simulink model "MCU_Input"  (R2022b)
settings: Solver=FixedStepDiscrete  StartTime=0.0  StopTime=10.0  FixedStep=1e-4  RelTol=1e-3
values from neighbouring files (symbols this model uses):
  C_ADC_Acc1Offset_i32 = 0.0    [MCU_Input_Sldd.sldd]    (also in MCU_Input_Sldd_objects.m = myPackage.Parameter)
  C_ADC_BrakeOffset_i32 = 0.0    [MCU_Input_Sldd.sldd]    (also in MCU_Input_Sldd_objects.m = myPackage.Parameter)
  C_ADC_HSTempGain_f32 = 0.0    [MCU_Input_Sldd.sldd]    (also in MCU_Input_Sldd_objects.m = myPackage.Parameter)
  C_ADC_HSTempOffset_i32 = 0.0    [MCU_Input_Sldd.sldd]    (also in MCU_Input_Sldd_objects.m = myPackage.Parameter)
  C_ADC_IdcOffset_i32 = 0.0    [MCU_Input_Sldd.sldd]    (also in MCU_Input_Sldd_objects.m = myPackage.Parameter)
  C_ADC_IGBTTable_i16 = 0.0    [MCU_Input_Sldd.sldd]    (also in MCU_Input_Sldd_objects.m = myPackage.Parameter)
  C_ADC_IGBTTempGain_f32 = 0.0    [MCU_Input_Sldd.sldd]    (also in MCU_Input_Sldd_objects.m = myPackage.Parameter)
  C_ADC_IGBTTempOffset_i32 = 0.0    [MCU_Input_Sldd.sldd]    (also in MCU_Input_Sldd_objects.m = myPackage.Parameter)
  C_ADC_MotorTemp1Gain_f32 = 0.0    [MCU_Input_Sldd.sldd]    (also in MCU_Input_Sldd_objects.m = myPackage.Parameter)
  C_ADC_MotorTemp1Offset_i32 = 0.0    [MCU_Input_Sldd.sldd]    (also in MCU_Input_Sldd_objects.m = myPackage.Parameter)
  C_ADC_MotorTempTable_i16 = 0.0    [MCU_Input_Sldd.sldd]    (also in MCU_Input_Sldd_objects.m = myPackage.Parameter)
  C_ADC_P12VOffset_i32 = 0.0    [MCU_Input_Sldd.sldd]    (also in MCU_Input_Sldd_objects.m = myPackage.Parameter)
  C_ADC_P15VOffset_i32 = 0.0    [MCU_Input_Sldd.sldd]    (also in MCU_Input_Sldd_objects.m = myPackage.Parameter)
  C_ADC_P5VOffset_i32 = 0.0    [MCU_Input_Sldd.sldd]    (also in MCU_Input_Sldd_objects.m = myPackage.Parameter)
  C_DCCurrent_DrvCoeff_f32 = 0.0    [MCU_Input_Sldd.sldd]    (also in MCU_Input_Sldd_objects.m = myPackage.Parameter)
  C_DCCurrent_GenCoeff_f32 = 0.0    [MCU_Input_Sldd.sldd]    (also in MCU_Input_Sldd_objects.m = myPackage.Parameter)
  C_Encoder_CurrentAdder_f32 = 0.0    [MCU_Input_Sldd.sldd]    (also in MCU_Input_Sldd_objects.m = myPackage.Parameter)
  C_Encoder_WaitTime_f32 = 0.0    [MCU_Input_Sldd.sldd]    (also in MCU_Input_Sldd_objects.m = myPackage.Parameter)
  C_Input_EncErr_u8 = 0.0    [MCU_Input_Sldd.sldd]    (also in MCU_Input_Sldd_objects.m = myPackage.Parameter)
  C_Rotate_RotateBits_u8 = 0.0    [MCU_Input_Sldd.sldd]    (also in MCU_Input_Sldd_objects.m = myPackage.Parameter)
  C_Rotate_SetAngle_u16 = 0.0    [MCU_Input_Sldd.sldd]    (also in MCU_Input_Sldd_objects.m = myPackage.Parameter)
  C_Rotate_SetAngleFlg_u8 = 0.0    [MCU_Input_Sldd.sldd]    (also in MCU_Input_Sldd_objects.m = myPackage.Parameter)
  C_SelfCheck_AvgCntSet_u16 = 0.0    [MCU_Input_Sldd.sldd]    (also in MCU_Input_Sldd_objects.m = myPackage.Parameter)
  C_SelfCheck_DelayTimeSet_u16 = 0.0    [MCU_Input_Sldd.sldd]    (also in MCU_Input_Sldd_objects.m = myPackage.Parameter)
  C_SelfCheck_IaoffsetDownLimt_u16 = 0.0    [MCU_Input_Sldd.sldd]    (also in MCU_Input_Sldd_objects.m = myPackage.Parameter)
  C_SelfCheck_IaoffsetUpLimt_u16 = 0.0    [MCU_Input_Sldd.sldd]    (also in MCU_Input_Sldd_objects.m = myPackage.Parameter)
  C_SelfCheck_IboffsetDownLimt_u16 = 0.0    [MCU_Input_Sldd.sldd]    (also in MCU_Input_Sldd_objects.m = myPackage.Parameter)
  C_SelfCheck_IboffsetUpLimt_u16 = 0.0    [MCU_Input_Sldd.sldd]    (also in MCU_Input_Sldd_objects.m = myPackage.Parameter)
  C_SelfCheck_IcoffsetDownLimt_u16 = 0.0    [MCU_Input_Sldd.sldd]    (also in MCU_Input_Sldd_objects.m = myPackage.Parameter)
  C_SelfCheck_IcoffsetUpLimt_u16 = 0.0    [MCU_Input_Sldd.sldd]    (also in MCU_Input_Sldd_objects.m = myPackage.Parameter)
  C_SelfCheck_OffsetUnCal_u8 = 0.0    [MCU_Input_Sldd.sldd]    (also in MCU_Input_Sldd_objects.m = myPackage.Parameter)
undefined symbols (not defined in the file or in its folder): AB_SAMPLE, ABC_SAMPLE, AC_SAMPLE, ANALOG, BC_SAMPLE, cAgeingMode, cParaRecogMode, cVvvfOpenMode, ParamCfg_AdAcc1K_u16, ParamCfg_AdBrakeK_u16, ParamCfg_AdIaK_u16, ParamCfg_AdIbK_u16, ParamCfg_AdIcK_u16, ParamCfg_AdKeyK_u16, ParamCfg_AdP12vK_u16, ParamCfg_AdP15vK_u16, ParamCfg_AdP5vK_u16, ParamCfg_AdUdcK_u16, ParamCfg_AdVonK_u16, ParamCfg_Avgcnt_u16, ParamCfg_BaseCur_u16, ParamCfg_BaseUdc_u16, ParamCfg_CommandSource_u16, ParamCfg_MaxSpeed_u16, ParamCfg_MotorNp_u16, ParamCfg_PosInit_u16, ParamCfg_PowerMax_u16, ParamCfg_PwmFreqLow_u16, ParamCfg_RotateDir_u16, ParamCfg_RotateNp_u16, ParamCfg_SampleMode_u16, ParamCfg_SensorSpeed_u16, ParamCfg_SmoPllKi_u16, ParamCfg_SmoPllKp_u16, ParamCfg_Stage_u16, ParamCfg_ThetaGain_u16, ParamCfg_UdcDefValue_u16, POWER_ON, STANDBY
libraries: simulink x41, YS_UserDefined_Library x4
(part 3 of 5)

== system MCU_Input/Input_100us/DCCurrent_100us/DcCurrentCal/FirstOrder_LPF_Calc ==
  Xn : Inport
  Add : Sum
  Compare To Constant : simulink/Logic and Bit Operations/Compare To Constant  relop=<  const=1  OutDataTypeStr=boolean
  Constant : Constant  Value=0.01  OutDataTypeStr=single
  Constant1 : Constant  OutDataTypeStr=single
  Minus : Sum  Inputs=+-
  Minus1 : Sum  Inputs=-+
  Product : Product
  Product1 : Product
  Switch : Switch  Criteria=u2 > Threshold  SaturateOnIntegerOverflow=off  InputSameDT=off
  Unit Delay : UnitDelay  SampleTime=-1  HasFrameUpgradeWarning=on
  Yn : Outport
  wires:
  Switch/1 -> Unit Delay/1, Yn/1
  Unit Delay/1 -> Product1/2, Minus/2  "Yn_1"
  Xn/1 -> Minus/1, Product/1, Switch/1
  Minus/1 -> Compare To Constant/1
  Compare To Constant/1 -> Switch/2
  Constant/1 -> Minus1/1, Product/2
  Product/1 -> Add/1
  Constant1/1 -> Minus1/2
  Minus1/1 -> Product1/1
  Product1/1 -> Add/2
  Add/1 -> Switch/3

== system MCU_Input/Input_100us/DCCurrent_100us/DcCurrentCal/RandCurGen ==
  Add : Sum
  Compare To Constant : simulink/Logic and Bit Operations/Compare To Constant  relop=>=  const=41  OutDataTypeStr=boolean
  Constant : Constant  OutDataTypeStr=uint8
  RandCurArray : Constant  Value=[1, 7, 5, 2, 4, 5, 8, 6, 3, 5, 1, 10, 7, 5, 0, 2, 4, 5, 8, 6, 3, 8, 6, 3, 5, 1, 10, 7, 5, 2, 10, 7, 5, 0, 2, 4, 5, 8, 6, 3, 8]  OutDataTypeStr=uint16
  Selector : Selector  InputPortWidth=41  IndexOptions=Index vector (port)  Indices=[1 3]  OutputSizes=1
  Switch : Switch  Criteria=u2 ~= 0  SaturateOnIntegerOverflow=off  InputSameDT=off
  Unit Delay : UnitDelay  SampleTime=-1  HasFrameUpgradeWarning=on
  RandCur : Outport
  wires:
  Add/1 -> Selector/2, Unit Delay/1
  Constant/1 -> Add/1, Switch/1
  Compare To Constant/1 -> Switch/2
  Unit Delay/1 -> Switch/3, Compare To Constant/1
  Switch/1 -> Add/2
  RandCurArray/1 -> Selector/1
  Selector/1 -> RandCur/1

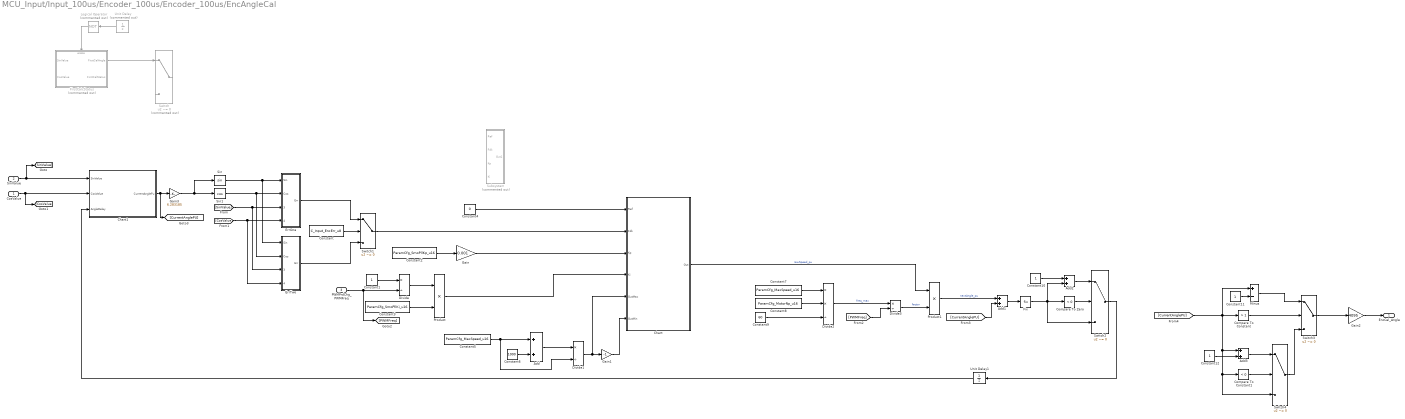
== system MCU_Input/Input_100us/Encoder_100us/Encoder_100us/EncAngleCal ==
  CosValue : Inport
  SinValue : Inport  Port=2
  PWMPrdChg_PWMFreq : Inport  Port=3
  Add : Sum
  Add1 : Sum  OutDataTypeStr=single
  Add2 : Sum
  Add3 : Sum
  Chart : Stateflow chart  TreatAsAtomicUnit=on
  Chart1 : Stateflow chart  TreatAsAtomicUnit=on
  Compare To Constant : simulink/Logic and Bit Operations/Compare To Constant  relop=>  const=1  OutDataTypeStr=boolean
  Compare To Constant1 : simulink/Logic and Bit Operations/Compare To Constant  relop=<  const=0  OutDataTypeStr=boolean
  Compare To Zero : simulink/Logic and Bit Operations/Compare To Zero  relop=<  OutDataTypeStr=boolean
  Constant : Constant  Value=C_Input_EncErr_u8
  Constant{1,10..12} (4 alike) : Constant  OutDataTypeStr=single
  Constant2 : Constant  Value=ParamCfg_SmoPllKp_u16
  Constant3 : Constant  Value=ParamCfg_SmoPllKi_u16
  Constant4 : Constant  Value=0  OutDataTypeStr=single
  Constant5 : Constant  Value=ParamCfg_MaxSpeed_u16
  Constant6 : Constant  Value=1000  OutDataTypeStr=single
  Constant7 : Constant  Value=ParamCfg_MaxSpeed_u16
  Constant8 : Constant  Value=ParamCfg_MotorNp_u16
  Constant9 : Constant  Value=60  OutDataTypeStr=single
  Divide : Product  Inputs=*/  OutDataTypeStr=single
  Divide1 : Product  Inputs=*/
  Divide2 : Product  Inputs=**/
  Divide3 : Product  Inputs=*/
  ErrOne : Subsystem
  ErrTwo : Subsystem
  FirstCalcStatus : Subsystem  Commented=on
  Fix : Rounding  Operator=fix
  Gain : Gain  Gain=0.001  ParamDataTypeStr=single  OutDataTypeStr=single
  Gain1 : Gain  Gain=-1  ParamDataTypeStr=single  OutDataTypeStr=single
  Gain2 : Gain  Gain=4095  ParamDataTypeStr=uint16  OutDataTypeStr=uint16
  Gain3 : Gain  Gain=6.283185  ParamDataTypeStr=single  OutDataTypeStr=single
      settings: AttributesFormatString=%<Gain>
  Logical Operator : Logic  Commented=on  Operator=NOT  AllPortsSameDT=off  OutDataTypeStr=boolean
  Minus : Sum  Inputs=+-
  Product : Product
  Product1 : Product
  Sin : Trigonometry
  Sin1 : Trigonometry  Operator=cos
  Subsystem : Subsystem  Commented=on
  Switch : Switch  Commented=on  Criteria=u2 ~= 0  SaturateOnIntegerOverflow=off  InputSameDT=off
  Switch{1..4} (4 alike) : Switch  Criteria=u2 ~= 0  SaturateOnIntegerOverflow=off  InputSameDT=off
  Unit Delay : UnitDelay  Commented=on  SampleTime=-1  HasFrameUpgradeWarning=on
  Unit Delay1 : UnitDelay  SampleTime=-1  HasFrameUpgradeWarning=on
  EncCal_Angle : Outport
  wires:
  SinValue/1 -> [SinValue], Chart1/1(SinValue)
  CosValue/1 -> Chart1/2(CosValue), [CosValue]
  Chart1/1(CurrentAnglePu) -> [CurrentAnglePU], Gain3/1
  Unit Delay/1 -> Logical Operator/1
  Logical Operator/1 -> FirstCalcStatus/Enable
  FirstCalcStatus/1(FirstCalAngle) -> Switch/1
  Sin/1 -> ErrTwo/1(Sin), ErrOne/1(Sin)
  Sin1/1 -> ErrTwo/2(Cos), ErrOne/2(Cos)
  [SinValue] -> ErrTwo/3(SinValue), ErrOne/3(SinValue)
  [CosValue] -> ErrTwo/4(CosValue), ErrOne/4(CosValue)
  Constant/1 -> Switch1/2
  ErrOne/1(Err) -> Switch1/1
  ErrTwo/1(Err) -> Switch1/3
  PWMPrdChg_PWMFreq/1 -> [PWMFreq], Divide/2
  Constant1/1 -> Divide/1
  Constant2/1 -> Gain/1
  Divide/1 -> Product/1
  Constant3/1 -> Product/2
  Constant4/1 -> Chart/1(Ref)
  Switch1/1 -> Chart/2(Fdk)
  Gain/1 -> Chart/3(Kp)
  Product/1 -> Chart/4(Ki)
  Constant6/1 -> Add/2
  Divide1/1 -> Chart/5(OutMax), Gain1/1
  Constant5/1 -> Add/1, Divide1/2
  Add/1 -> Divide1/1
  Gain1/1 -> Chart/6(OutMin)
  Chart/1(Out) -> Product1/1  "rawSpeed_pu"
  Constant7/1 -> Divide2/1
  Constant8/1 -> Divide2/2
  Constant9/1 -> Divide2/3
  Divide2/1 -> Divide3/1  "freq_max"
  [PWMFreq] -> Divide3/2
  Divide3/1 -> Product1/2  "factor"
  Product1/1 -> Add1/1  "nextAngle_pu"
  Add1/1 -> Fix/1
  Unit Delay1/1 -> Chart1/3(AngleDelay)
  Fix/1 -> Add2/2, Switch2/3, Compare To Zero/1
  Compare To Zero/1 -> Switch2/2
  Add2/1 -> Switch2/1
  Constant10/1 -> Add2/1
  [CurrentAnglePU] -> Compare To Constant/1, Switch4/3, Compare To Constant1/1, Add3/1, Minus/1
  Compare To Constant/1 -> Switch3/2
  Constant11/1 -> Minus/2
  Minus/1 -> Switch3/1
  Switch4/1 -> Switch3/3
  Compare To Constant1/1 -> Switch4/2
  Add3/1 -> Switch4/1
  Constant12/1 -> Add3/2
  Switch3/1 -> Gain2/1
  Gain2/1 -> EncCal_Angle/1
  Gain3/1 -> Sin/1, Sin1/1
  [CurrentAnglePU] -> Add1/2
  Switch2/1 -> Unit Delay1/1

== system MCU_Input/Input_100us/Encoder_100us/Encoder_100us/EncCalibCal/AmpCos ==
  CosRaw : Inport  OutDataTypeStr=uint16  PortDimensions=1
  f : TriggerPort  TriggerType=function-call  VariantControl=(inherit)
      settings: CopyFcn=Stateflow.SLINSF.SimulinkMan.removeBlockPreDeleteFcn  PreDeleteFcn=Stateflow.SLINSF.SimulinkMan.unsafePredeleteFcn
  Data Store Read : DataStoreRead  DataStoreName=CosMin  IndexOptions=Index vector (dialog)  Indices=1  OutputSizes=1
  Data Store Read1 : DataStoreRead  DataStoreName=CosMax  IndexOptions=Index vector (dialog)  Indices=1  OutputSizes=1
  Data Store Write : DataStoreWrite  DataStoreName=CosMax  IndexOptions=Index vector (dialog)  Indices=1  OutputSizes=1
  Data Store Write1 : DataStoreWrite  DataStoreName=CosMin  IndexOptions=Index vector (dialog)  Indices=1  OutputSizes=1
  Gain : Gain  Gain=0.5  ParamDataTypeStr=single  OutDataTypeStr=single
  Minus : Sum  Inputs=+-
  Relational Operator : RelationalOperator  Operator=>  OutDataTypeStr=boolean  RndMeth=Simplest  InputSameDT=off
  Relational Operator1 : RelationalOperator  Operator=<  OutDataTypeStr=boolean  RndMeth=Simplest  InputSameDT=off
  Switch : Switch  Criteria=u2 ~= 0  SaturateOnIntegerOverflow=off  InputSameDT=off
  Switch1 : Switch  Criteria=u2 ~= 0  SaturateOnIntegerOverflow=off  InputSameDT=off
  CosAmp : Outport  OutDataTypeStr=single
  wires:
  CosRaw/1 -> Switch1/1, Relational Operator1/1, Switch/1, Relational Operator/1
  Data Store Read1/1 -> Switch/3, Relational Operator/2
  Relational Operator/1 -> Switch/2
  Switch/1 -> Minus/1, Data Store Write/1
  Data Store Read/1 -> Switch1/3, Relational Operator1/2
  Relational Operator1/1 -> Switch1/2
  Switch1/1 -> Minus/2, Data Store Write1/1
  Minus/1 -> Gain/1
  Gain/1 -> CosAmp/1

== system MCU_Input/Input_100us/Encoder_100us/Encoder_100us/EncCalibCal/AmpSin ==
  SinRaw : Inport  OutDataTypeStr=uint16  PortDimensions=1
  f : TriggerPort  TriggerType=function-call  VariantControl=(inherit)
      settings: CopyFcn=Stateflow.SLINSF.SimulinkMan.removeBlockPreDeleteFcn  PreDeleteFcn=Stateflow.SLINSF.SimulinkMan.unsafePredeleteFcn
  Data Store Read : DataStoreRead  DataStoreName=SinMin  IndexOptions=Index vector (dialog)  Indices=1  OutputSizes=1
  Data Store Read1 : DataStoreRead  DataStoreName=SinMax  IndexOptions=Index vector (dialog)  Indices=1  OutputSizes=1
  Data Store Write : DataStoreWrite  DataStoreName=SinMax  IndexOptions=Index vector (dialog)  Indices=1  OutputSizes=1
  Data Store Write1 : DataStoreWrite  DataStoreName=SinMin  IndexOptions=Index vector (dialog)  Indices=1  OutputSizes=1
  Gain : Gain  Gain=0.5  ParamDataTypeStr=single  OutDataTypeStr=single
  Minus : Sum  Inputs=+-  AccumDataTypeStr=uint16  OutDataTypeStr=uint16
  Relational Operator : RelationalOperator  Operator=>  OutDataTypeStr=boolean  RndMeth=Simplest  InputSameDT=off
  Relational Operator1 : RelationalOperator  Operator=<  OutDataTypeStr=boolean  RndMeth=Simplest  InputSameDT=off
  Switch : Switch  Criteria=u2 ~= 0  SaturateOnIntegerOverflow=off  InputSameDT=off
  Switch1 : Switch  Criteria=u2 ~= 0  SaturateOnIntegerOverflow=off  InputSameDT=off
  SinAmp : Outport  OutDataTypeStr=single  PortDimensions=1
  wires:
  SinRaw/1 -> Switch1/1, Relational Operator1/1, Switch/1, Relational Operator/1
  Data Store Read1/1 -> Switch/3, Relational Operator/2
  Relational Operator/1 -> Switch/2
  Switch/1 -> Minus/1, Data Store Write/1
  Data Store Read/1 -> Switch1/3, Relational Operator1/2
  Relational Operator1/1 -> Switch1/2
  Switch1/1 -> Minus/2, Data Store Write1/1
  Minus/1 -> Gain/1
  Gain/1 -> SinAmp/1

== system MCU_Input/Input_100us/Encoder_100us/Encoder_100us/EncCalibCal1/AmpCos ==
  CosRaw : Inport  OutDataTypeStr=uint16  PortDimensions=1
  f : TriggerPort  TriggerType=function-call  VariantControl=(inherit)
      settings: CopyFcn=Stateflow.SLINSF.SimulinkMan.removeBlockPreDeleteFcn  PreDeleteFcn=Stateflow.SLINSF.SimulinkMan.unsafePredeleteFcn
  Data Store Read : DataStoreRead  DataStoreName=CosMin  IndexOptions=Index vector (dialog)  Indices=1  OutputSizes=1
  Data Store Read1 : DataStoreRead  DataStoreName=CosMax  IndexOptions=Index vector (dialog)  Indices=1  OutputSizes=1
  Data Store Write : DataStoreWrite  DataStoreName=CosMax  IndexOptions=Index vector (dialog)  Indices=1  OutputSizes=1
  Data Store Write1 : DataStoreWrite  DataStoreName=CosMin  IndexOptions=Index vector (dialog)  Indices=1  OutputSizes=1
  Gain : Gain  Gain=0.5  ParamDataTypeStr=single  OutDataTypeStr=single
  Minus : Sum  Inputs=+-
  Relational Operator : RelationalOperator  Operator=>  OutDataTypeStr=boolean  RndMeth=Simplest  InputSameDT=off
  Relational Operator1 : RelationalOperator  Operator=<  OutDataTypeStr=boolean  RndMeth=Simplest  InputSameDT=off
  Switch : Switch  Criteria=u2 ~= 0  SaturateOnIntegerOverflow=off  InputSameDT=off
  Switch1 : Switch  Criteria=u2 ~= 0  SaturateOnIntegerOverflow=off  InputSameDT=off
  CosAmp : Outport  OutDataTypeStr=single
  wires:
  CosRaw/1 -> Switch1/1, Relational Operator1/1, Switch/1, Relational Operator/1
  Data Store Read1/1 -> Switch/3, Relational Operator/2
  Relational Operator/1 -> Switch/2
  Switch/1 -> Minus/1, Data Store Write/1
  Data Store Read/1 -> Switch1/3, Relational Operator1/2
  Relational Operator1/1 -> Switch1/2
  Switch1/1 -> Minus/2, Data Store Write1/1
  Minus/1 -> Gain/1
  Gain/1 -> CosAmp/1

== system MCU_Input/Input_100us/Encoder_100us/Encoder_100us/EncCalibCal1/AmpSin ==
  SinRaw : Inport  OutDataTypeStr=uint16  PortDimensions=1
  f : TriggerPort  TriggerType=function-call  VariantControl=(inherit)
      settings: CopyFcn=Stateflow.SLINSF.SimulinkMan.removeBlockPreDeleteFcn  PreDeleteFcn=Stateflow.SLINSF.SimulinkMan.unsafePredeleteFcn
  Data Store Read : DataStoreRead  DataStoreName=SinMin  IndexOptions=Index vector (dialog)  Indices=1  OutputSizes=1
  Data Store Read1 : DataStoreRead  DataStoreName=SinMax  IndexOptions=Index vector (dialog)  Indices=1  OutputSizes=1
  Data Store Write : DataStoreWrite  DataStoreName=SinMax  IndexOptions=Index vector (dialog)  Indices=1  OutputSizes=1
  Data Store Write1 : DataStoreWrite  DataStoreName=SinMin  IndexOptions=Index vector (dialog)  Indices=1  OutputSizes=1
  Gain : Gain  Gain=0.5  ParamDataTypeStr=single  OutDataTypeStr=single
  Minus : Sum  Inputs=+-  AccumDataTypeStr=uint16  OutDataTypeStr=uint16
  Relational Operator : RelationalOperator  Operator=>  OutDataTypeStr=boolean  RndMeth=Simplest  InputSameDT=off
  Relational Operator1 : RelationalOperator  Operator=<  OutDataTypeStr=boolean  RndMeth=Simplest  InputSameDT=off
  Switch : Switch  Criteria=u2 ~= 0  SaturateOnIntegerOverflow=off  InputSameDT=off
  Switch1 : Switch  Criteria=u2 ~= 0  SaturateOnIntegerOverflow=off  InputSameDT=off
  SinAmp : Outport  OutDataTypeStr=single  PortDimensions=1
  wires:
  SinRaw/1 -> Switch1/1, Relational Operator1/1, Switch/1, Relational Operator/1
  Data Store Read1/1 -> Switch/3, Relational Operator/2
  Relational Operator/1 -> Switch/2
  Switch/1 -> Minus/1, Data Store Write/1
  Data Store Read/1 -> Switch1/3, Relational Operator1/2
  Relational Operator1/1 -> Switch1/2
  Switch1/1 -> Minus/2, Data Store Write1/1
  Minus/1 -> Gain/1
  Gain/1 -> SinAmp/1

== system MCU_Input/Input_100us/Encoder_100us/Encoder_100us/EncCalibCal2/AmpCos ==
  CosRaw : Inport  OutDataTypeStr=uint16  PortDimensions=1
  f : TriggerPort  TriggerType=function-call  VariantControl=(inherit)
      settings: CopyFcn=Stateflow.SLINSF.SimulinkMan.removeBlockPreDeleteFcn  PreDeleteFcn=Stateflow.SLINSF.SimulinkMan.unsafePredeleteFcn
  Data Store Read : DataStoreRead  DataStoreName=CosMin  IndexOptions=Index vector (dialog)  Indices=1  OutputSizes=1
  Data Store Read1 : DataStoreRead  DataStoreName=CosMax  IndexOptions=Index vector (dialog)  Indices=1  OutputSizes=1
  Data Store Write : DataStoreWrite  DataStoreName=CosMax  IndexOptions=Index vector (dialog)  Indices=1  OutputSizes=1
  Data Store Write1 : DataStoreWrite  DataStoreName=CosMin  IndexOptions=Index vector (dialog)  Indices=1  OutputSizes=1
  Gain : Gain  Gain=0.5  ParamDataTypeStr=single  OutDataTypeStr=single
  Minus : Sum  Inputs=+-
  Relational Operator : RelationalOperator  Operator=>  OutDataTypeStr=boolean  RndMeth=Simplest  InputSameDT=off
  Relational Operator1 : RelationalOperator  Operator=<  OutDataTypeStr=boolean  RndMeth=Simplest  InputSameDT=off
  Switch : Switch  Criteria=u2 ~= 0  SaturateOnIntegerOverflow=off  InputSameDT=off
  Switch1 : Switch  Criteria=u2 ~= 0  SaturateOnIntegerOverflow=off  InputSameDT=off
  CosAmp : Outport  OutDataTypeStr=single
  wires:
  Gain/1 -> CosAmp/1
  Minus/1 -> Gain/1
  Switch1/1 -> Data Store Write1/1, Minus/2
  Relational Operator1/1 -> Switch1/2
  Data Store Read/1 -> Relational Operator1/2, Switch1/3
  Switch/1 -> Data Store Write/1, Minus/1
  Relational Operator/1 -> Switch/2
  Data Store Read1/1 -> Relational Operator/2, Switch/3
  CosRaw/1 -> Relational Operator/1, Switch/1, Relational Operator1/1, Switch1/1

== system MCU_Input/Input_100us/Encoder_100us/Encoder_100us/EncCalibCal2/AmpSin ==
  SinRaw : Inport  OutDataTypeStr=uint16  PortDimensions=1
  f : TriggerPort  TriggerType=function-call  VariantControl=(inherit)
      settings: CopyFcn=Stateflow.SLINSF.SimulinkMan.removeBlockPreDeleteFcn  PreDeleteFcn=Stateflow.SLINSF.SimulinkMan.unsafePredeleteFcn
  Data Store Read : DataStoreRead  DataStoreName=SinMin  IndexOptions=Index vector (dialog)  Indices=1  OutputSizes=1
  Data Store Read1 : DataStoreRead  DataStoreName=SinMax  IndexOptions=Index vector (dialog)  Indices=1  OutputSizes=1
  Data Store Write : DataStoreWrite  DataStoreName=SinMax  IndexOptions=Index vector (dialog)  Indices=1  OutputSizes=1
  Data Store Write1 : DataStoreWrite  DataStoreName=SinMin  IndexOptions=Index vector (dialog)  Indices=1  OutputSizes=1
  Gain : Gain  Gain=0.5  ParamDataTypeStr=single  OutDataTypeStr=single
  Minus : Sum  Inputs=+-  AccumDataTypeStr=uint16  OutDataTypeStr=uint16
  Relational Operator : RelationalOperator  Operator=>  OutDataTypeStr=boolean  RndMeth=Simplest  InputSameDT=off
  Relational Operator1 : RelationalOperator  Operator=<  OutDataTypeStr=boolean  RndMeth=Simplest  InputSameDT=off
  Switch : Switch  Criteria=u2 ~= 0  SaturateOnIntegerOverflow=off  InputSameDT=off
  Switch1 : Switch  Criteria=u2 ~= 0  SaturateOnIntegerOverflow=off  InputSameDT=off
  SinAmp : Outport  OutDataTypeStr=single  PortDimensions=1
  wires:
  Gain/1 -> SinAmp/1
  Minus/1 -> Gain/1
  Switch1/1 -> Data Store Write1/1, Minus/2
  Relational Operator1/1 -> Switch1/2
  Data Store Read/1 -> Relational Operator1/2, Switch1/3
  Switch/1 -> Data Store Write/1, Minus/1
  Relational Operator/1 -> Switch/2
  Data Store Read1/1 -> Relational Operator/2, Switch/3
  SinRaw/1 -> Relational Operator/1, Switch/1, Relational Operator1/1, Switch1/1

== system MCU_Input/Input_100us/Rotate_100us/RotateCalc/En ==
  EncCal_Angle : Inport
  MaxPos : Inport  Port=2
  MaxBorder : Inport  Port=3
  SelfCheckNoOverFlag : Inport  Port=4
  Enable : EnablePort
  Chart : Stateflow chart  TreatAsAtomicUnit=on
      settings: PortSchema="{\"entries\":[{\"content\":{\"sides\":[{\"content\":{\"connectorIds\":[\"In1\",\"In2\",\"In3\",\"In4\"]},\"type\":\"ConnectorPlacement.EquallySpacedRectSide\",\"uuid\":\"0d90a98d-d583-4b9f-a969-614b0a02b038\"},{\"content\":{\"connectorIds\":[\"Out1\",\"Out3\",\"Out4\",\"Out2\"],\"side\":\"RIGHT\"},\"type\":\"ConnectorPlacement.EquallySpacedRectSide\",\"uuid\":\"d1b62b16-d68a-4bf6-969a-465c170d794b\"},{\"content\":{\"connectorIds\":[],\"side\":\"TOP\"},\"type\":\"ConnectorPlacement.EquallySpacedRectSide\",\"uuid\":\"9c0d32d9-820c-46ff-a5ee-f3b4296aa9ac\"}]},\"type\":\"ConnectorPlacement.EquallySpacedConnector\",\"uuid\":\"994551a6-94d2-4e31-9518-9a38e84d14a2\"}],\"packageUris\":[\"http://schema.mathworks.com/mf0/Connector/R2020b\"],\"version\":\"1.0\"}"
  PosStart : Outport
  PosNew : Outport  Port=2
  PosAce : Outport  Port=3
  PosDelt : Outport  Port=4
  wires:
  SelfCheckNoOverFlag/1 -> Chart/4(SelfCheckNoOverFlag)
  MaxBorder/1 -> Chart/3(MaxBorder)
  Chart/3(PosNew) -> PosNew/1
  Chart/1(PosStart) -> PosStart/1
  EncCal_Angle/1 -> Chart/1(EncCal_Angle)
  Chart/2(PosDelt) -> PosDelt/1
  MaxPos/1 -> Chart/2(MaxPos)
  Chart/4(PosAce) -> PosAce/1

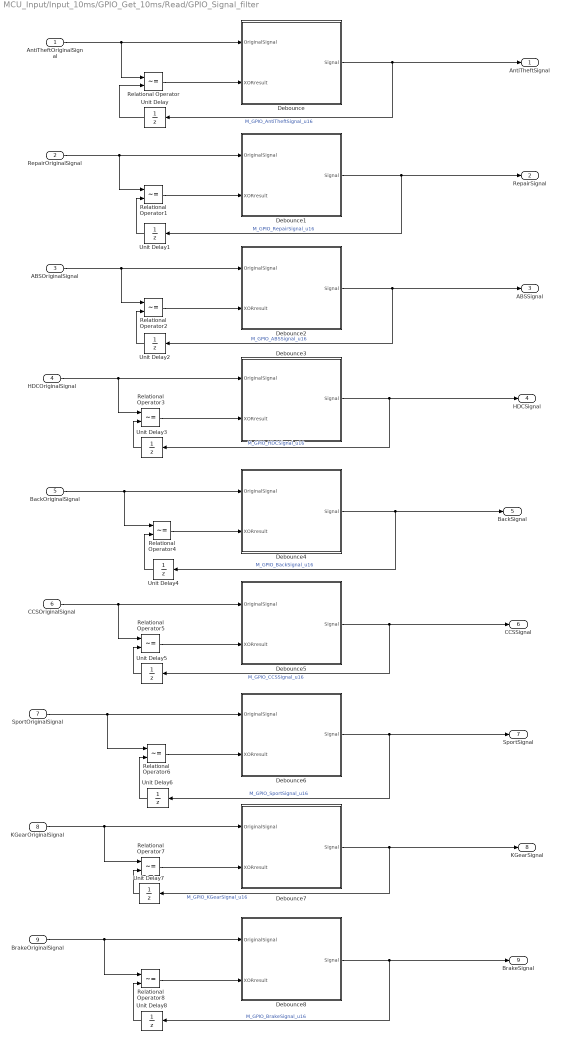
== system MCU_Input/Input_10ms/GPIO_Get_10ms/Read/GPIO_Signal_filter ==
  AntiTheftOriginalSignal : Inport
  RepairOriginalSignal : Inport  Port=2
  ABSOriginalSignal : Inport  Port=3
  HDCOriginalSignal : Inport  Port=4
  BackOriginalSignal : Inport  Port=5
  CCSOriginalSignal : Inport  Port=6
  SportOriginalSignal : Inport  Port=7
  KGearOriginalSignal : Inport  Port=8
  BrakeOriginalSignal : Inport  Port=9
  Debounce : Stateflow chart  TreatAsAtomicUnit=on
      settings: PortSchema="{\"entries\":[{\"content\":{\"sides\":[{\"content\":{\"connectorIds\":[\"In2\",\"In1\"]},\"type\":\"ConnectorPlacement.EquallySpacedRectSide\",\"uuid\":\"d2b7c253-4fee-4fc5-8521-157532493a48\"},{\"content\":{\"connectorIds\":[\"Out1\"],\"side\":\"RIGHT\"},\"type\":\"ConnectorPlacement.EquallySpacedRectSide\",\"uuid\":\"f5d0f306-fb12-43b3-9238-7da744c14b58\"},{\"content\":{\"connectorIds\":[],\"side\":\"TOP\"},\"type\":\"ConnectorPlacement.EquallySpacedRectSide\",\"uuid\":\"b4769129-7cf8-400e-82ef-329dd2aed5b0\"}]},\"type\":\"ConnectorPlacement.EquallySpacedConnector\",\"uuid\":\"7589d83e-379f-48f3-ae77-782c8af0c58b\"}],\"packageUris\":[\"http://schema.mathworks.com/mf0/Connector/R2020b\"],\"version\":\"1.0\"}"
  Debounce1 : Stateflow chart  TreatAsAtomicUnit=on
      settings: PortSchema="{\"entries\":[{\"content\":{\"sides\":[{\"content\":{\"connectorIds\":[\"In2\",\"In1\"]},\"type\":\"ConnectorPlacement.EquallySpacedRectSide\",\"uuid\":\"d2b7c253-4fee-4fc5-8521-157532493a48\"},{\"content\":{\"connectorIds\":[\"Out1\"],\"side\":\"RIGHT\"},\"type\":\"ConnectorPlacement.EquallySpacedRectSide\",\"uuid\":\"f5d0f306-fb12-43b3-9238-7da744c14b58\"},{\"content\":{\"connectorIds\":[],\"side\":\"TOP\"},\"type\":\"ConnectorPlacement.EquallySpacedRectSide\",\"uuid\":\"b4769129-7cf8-400e-82ef-329dd2aed5b0\"}]},\"type\":\"ConnectorPlacement.EquallySpacedConnector\",\"uuid\":\"7589d83e-379f-48f3-ae77-782c8af0c58b\"}],\"packageUris\":[\"http://schema.mathworks.com/mf0/Connector/R2020b\"],\"version\":\"1.0\"}"
  Debounce2 : Stateflow chart  TreatAsAtomicUnit=on
      settings: PortSchema="{\"entries\":[{\"content\":{\"sides\":[{\"content\":{\"connectorIds\":[\"In2\",\"In1\"]},\"type\":\"ConnectorPlacement.EquallySpacedRectSide\",\"uuid\":\"d2b7c253-4fee-4fc5-8521-157532493a48\"},{\"content\":{\"connectorIds\":[\"Out1\"],\"side\":\"RIGHT\"},\"type\":\"ConnectorPlacement.EquallySpacedRectSide\",\"uuid\":\"f5d0f306-fb12-43b3-9238-7da744c14b58\"},{\"content\":{\"connectorIds\":[],\"side\":\"TOP\"},\"type\":\"ConnectorPlacement.EquallySpacedRectSide\",\"uuid\":\"b4769129-7cf8-400e-82ef-329dd2aed5b0\"}]},\"type\":\"ConnectorPlacement.EquallySpacedConnector\",\"uuid\":\"7589d83e-379f-48f3-ae77-782c8af0c58b\"}],\"packageUris\":[\"http://schema.mathworks.com/mf0/Connector/R2020b\"],\"version\":\"1.0\"}"
  Debounce3 : Stateflow chart  TreatAsAtomicUnit=on
      settings: PortSchema="{\"entries\":[{\"content\":{\"sides\":[{\"content\":{\"connectorIds\":[\"In2\",\"In1\"]},\"type\":\"ConnectorPlacement.EquallySpacedRectSide\",\"uuid\":\"d2b7c253-4fee-4fc5-8521-157532493a48\"},{\"content\":{\"connectorIds\":[\"Out1\"],\"side\":\"RIGHT\"},\"type\":\"ConnectorPlacement.EquallySpacedRectSide\",\"uuid\":\"f5d0f306-fb12-43b3-9238-7da744c14b58\"},{\"content\":{\"connectorIds\":[],\"side\":\"TOP\"},\"type\":\"ConnectorPlacement.EquallySpacedRectSide\",\"uuid\":\"b4769129-7cf8-400e-82ef-329dd2aed5b0\"}]},\"type\":\"ConnectorPlacement.EquallySpacedConnector\",\"uuid\":\"7589d83e-379f-48f3-ae77-782c8af0c58b\"}],\"packageUris\":[\"http://schema.mathworks.com/mf0/Connector/R2020b\"],\"version\":\"1.0\"}"
  Debounce4 : Stateflow chart  TreatAsAtomicUnit=on
      settings: PortSchema="{\"entries\":[{\"content\":{\"sides\":[{\"content\":{\"connectorIds\":[\"In2\",\"In1\"]},\"type\":\"ConnectorPlacement.EquallySpacedRectSide\",\"uuid\":\"d2b7c253-4fee-4fc5-8521-157532493a48\"},{\"content\":{\"connectorIds\":[\"Out1\"],\"side\":\"RIGHT\"},\"type\":\"ConnectorPlacement.EquallySpacedRectSide\",\"uuid\":\"f5d0f306-fb12-43b3-9238-7da744c14b58\"},{\"content\":{\"connectorIds\":[],\"side\":\"TOP\"},\"type\":\"ConnectorPlacement.EquallySpacedRectSide\",\"uuid\":\"b4769129-7cf8-400e-82ef-329dd2aed5b0\"}]},\"type\":\"ConnectorPlacement.EquallySpacedConnector\",\"uuid\":\"7589d83e-379f-48f3-ae77-782c8af0c58b\"}],\"packageUris\":[\"http://schema.mathworks.com/mf0/Connector/R2020b\"],\"version\":\"1.0\"}"
  Debounce5 : Stateflow chart  TreatAsAtomicUnit=on
      settings: PortSchema="{\"entries\":[{\"content\":{\"sides\":[{\"content\":{\"connectorIds\":[\"In2\",\"In1\"]},\"type\":\"ConnectorPlacement.EquallySpacedRectSide\",\"uuid\":\"d2b7c253-4fee-4fc5-8521-157532493a48\"},{\"content\":{\"connectorIds\":[\"Out1\"],\"side\":\"RIGHT\"},\"type\":\"ConnectorPlacement.EquallySpacedRectSide\",\"uuid\":\"f5d0f306-fb12-43b3-9238-7da744c14b58\"},{\"content\":{\"connectorIds\":[],\"side\":\"TOP\"},\"type\":\"ConnectorPlacement.EquallySpacedRectSide\",\"uuid\":\"b4769129-7cf8-400e-82ef-329dd2aed5b0\"}]},\"type\":\"ConnectorPlacement.EquallySpacedConnector\",\"uuid\":\"7589d83e-379f-48f3-ae77-782c8af0c58b\"}],\"packageUris\":[\"http://schema.mathworks.com/mf0/Connector/R2020b\"],\"version\":\"1.0\"}"
  Debounce6 : Stateflow chart  TreatAsAtomicUnit=on
      settings: PortSchema="{\"entries\":[{\"content\":{\"sides\":[{\"content\":{\"connectorIds\":[\"In2\",\"In1\"]},\"type\":\"ConnectorPlacement.EquallySpacedRectSide\",\"uuid\":\"d2b7c253-4fee-4fc5-8521-157532493a48\"},{\"content\":{\"connectorIds\":[\"Out1\"],\"side\":\"RIGHT\"},\"type\":\"ConnectorPlacement.EquallySpacedRectSide\",\"uuid\":\"f5d0f306-fb12-43b3-9238-7da744c14b58\"},{\"content\":{\"connectorIds\":[],\"side\":\"TOP\"},\"type\":\"ConnectorPlacement.EquallySpacedRectSide\",\"uuid\":\"b4769129-7cf8-400e-82ef-329dd2aed5b0\"}]},\"type\":\"ConnectorPlacement.EquallySpacedConnector\",\"uuid\":\"7589d83e-379f-48f3-ae77-782c8af0c58b\"}],\"packageUris\":[\"http://schema.mathworks.com/mf0/Connector/R2020b\"],\"version\":\"1.0\"}"
  Debounce7 : Stateflow chart  TreatAsAtomicUnit=on
      settings: PortSchema="{\"entries\":[{\"content\":{\"sides\":[{\"content\":{\"connectorIds\":[\"In2\",\"In1\"]},\"type\":\"ConnectorPlacement.EquallySpacedRectSide\",\"uuid\":\"d2b7c253-4fee-4fc5-8521-157532493a48\"},{\"content\":{\"connectorIds\":[\"Out1\"],\"side\":\"RIGHT\"},\"type\":\"ConnectorPlacement.EquallySpacedRectSide\",\"uuid\":\"f5d0f306-fb12-43b3-9238-7da744c14b58\"},{\"content\":{\"connectorIds\":[],\"side\":\"TOP\"},\"type\":\"ConnectorPlacement.EquallySpacedRectSide\",\"uuid\":\"b4769129-7cf8-400e-82ef-329dd2aed5b0\"}]},\"type\":\"ConnectorPlacement.EquallySpacedConnector\",\"uuid\":\"7589d83e-379f-48f3-ae77-782c8af0c58b\"}],\"packageUris\":[\"http://schema.mathworks.com/mf0/Connector/R2020b\"],\"version\":\"1.0\"}"
  Debounce8 : Stateflow chart  TreatAsAtomicUnit=on
      settings: PortSchema="{\"entries\":[{\"content\":{\"sides\":[{\"content\":{\"connectorIds\":[\"In2\",\"In1\"]},\"type\":\"ConnectorPlacement.EquallySpacedRectSide\",\"uuid\":\"d2b7c253-4fee-4fc5-8521-157532493a48\"},{\"content\":{\"connectorIds\":[\"Out1\"],\"side\":\"RIGHT\"},\"type\":\"ConnectorPlacement.EquallySpacedRectSide\",\"uuid\":\"f5d0f306-fb12-43b3-9238-7da744c14b58\"},{\"content\":{\"connectorIds\":[],\"side\":\"TOP\"},\"type\":\"ConnectorPlacement.EquallySpacedRectSide\",\"uuid\":\"b4769129-7cf8-400e-82ef-329dd2aed5b0\"}]},\"type\":\"ConnectorPlacement.EquallySpacedConnector\",\"uuid\":\"7589d83e-379f-48f3-ae77-782c8af0c58b\"}],\"packageUris\":[\"http://schema.mathworks.com/mf0/Connector/R2020b\"],\"version\":\"1.0\"}"
  Relational Operator{,1..8} (9 alike) : RelationalOperator  Operator=~=  OutDataTypeStr=boolean  RndMeth=Simplest  InputSameDT=off
  Unit Delay{,1..8} (9 alike) : UnitDelay  SampleTime=-1  HasFrameUpgradeWarning=on
  AntiTheftSignal : Outport
  RepairSignal : Outport  Port=2
  ABSSignal : Outport  Port=3
  HDCSignal : Outport  Port=4
  BackSignal : Outport  Port=5
  CCSSignal : Outport  Port=6
  SportSignal : Outport  Port=7
  KGearSignal : Outport  Port=8
  BrakeSignal : Outport  Port=9
  wires:
  Debounce/1(Signal) -> Unit Delay/1, AntiTheftSignal/1  "M_GPIO_AntiTheftSignal_u16"
  AntiTheftOriginalSignal/1 -> Relational Operator/1, Debounce/2(OriginalSignal)
  Unit Delay/1 -> Relational Operator/2
  Relational Operator/1 -> Debounce/1(XORresult)
  Relational Operator1/1 -> Debounce1/1(XORresult)
  RepairOriginalSignal/1 -> Relational Operator1/1, Debounce1/2(OriginalSignal)
  Unit Delay1/1 -> Relational Operator1/2
  Debounce1/1(Signal) -> Unit Delay1/1, RepairSignal/1  "M_GPIO_RepairSignal_u16"
  Unit Delay2/1 -> Relational Operator2/2
  Debounce2/1(Signal) -> Unit Delay2/1, ABSSignal/1  "M_GPIO_ABSSignal_u16"
  Relational Operator2/1 -> Debounce2/1(XORresult)
  ABSOriginalSignal/1 -> Relational Operator2/1, Debounce2/2(OriginalSignal)
  HDCOriginalSignal/1 -> Relational Operator3/1, Debounce3/2(OriginalSignal)
  Relational Operator3/1 -> Debounce3/1(XORresult)
  Debounce3/1(Signal) -> Unit Delay3/1, HDCSignal/1  "M_GPIO_HDCSignal_u16"
  Unit Delay3/1 -> Relational Operator3/2
  BackOriginalSignal/1 -> Relational Operator4/1, Debounce4/2(OriginalSignal)
  Relational Operator4/1 -> Debounce4/1(XORresult)
  Debounce4/1(Signal) -> Unit Delay4/1, BackSignal/1  "M_GPIO_BackSignal_u16"
  Unit Delay4/1 -> Relational Operator4/2
  CCSOriginalSignal/1 -> Relational Operator5/1, Debounce5/2(OriginalSignal)
  Relational Operator5/1 -> Debounce5/1(XORresult)
  Debounce5/1(Signal) -> Unit Delay5/1, CCSSignal/1  "M_GPIO_CCSSignal_u16"
  Unit Delay5/1 -> Relational Operator5/2
  SportOriginalSignal/1 -> Relational Operator6/1, Debounce6/2(OriginalSignal)
  Relational Operator6/1 -> Debounce6/1(XORresult)
  Debounce6/1(Signal) -> Unit Delay6/1, SportSignal/1  "M_GPIO_SportSignal_u16"
  Unit Delay6/1 -> Relational Operator6/2
  KGearOriginalSignal/1 -> Relational Operator7/1, Debounce7/2(OriginalSignal)
  Relational Operator7/1 -> Debounce7/1(XORresult)
  Debounce7/1(Signal) -> Unit Delay7/1, KGearSignal/1  "M_GPIO_KGearSignal_u16"
  Unit Delay7/1 -> Relational Operator7/2
  BrakeOriginalSignal/1 -> Relational Operator8/1, Debounce8/2(OriginalSignal)
  Relational Operator8/1 -> Debounce8/1(XORresult)
  Unit Delay8/1 -> Relational Operator8/2
  Debounce8/1(Signal) -> Unit Delay8/1, BrakeSignal/1  "M_GPIO_BrakeSignal_u16"

== system MCU_Input/Input_100us/Encoder_100us/Encoder_100us/EncAngleCal/Chart/Limitation ==
  In : Inport
  Max : Inport  Port=2
  Min : Inport  Port=3
  f : TriggerPort  TriggerType=function-call  VariantControl=(inherit)
      settings: CopyFcn=Stateflow.SLINSF.SimulinkMan.removeBlockPreDeleteFcn  PreDeleteFcn=Stateflow.SLINSF.SimulinkMan.unsafePredeleteFcn
  Relational Operator : RelationalOperator  Operator=>  OutDataTypeStr=boolean  RndMeth=Simplest  InputSameDT=off
  Relational Operator1 : RelationalOperator  Operator=>  OutDataTypeStr=boolean  RndMeth=Simplest  InputSameDT=off
  Switch : Switch  Criteria=u2 ~= 0  SaturateOnIntegerOverflow=off  InputSameDT=off
  Switch1 : Switch  Criteria=u2 ~= 0  SaturateOnIntegerOverflow=off  InputSameDT=off
  OutLimit : Outport
  wires:
  In/1 -> Switch1/1, Relational Operator/1
  Max/1 -> Switch/1, Relational Operator1/1, Relational Operator/2
  Relational Operator/1 -> Switch/2
  Min/1 -> Switch1/3, Relational Operator1/2
  Relational Operator1/1 -> Switch1/2
  Switch1/1 -> Switch/3
  Switch/1 -> OutLimit/1

== system MCU_Input/Input_100us/Encoder_100us/Encoder_100us/EncAngleCal/ErrOne ==
  Sin : Inport
  Cos : Inport  Port=2
  SinValue : Inport  Port=3
  CosValue : Inport  Port=4
  Minus : Sum  Inputs=+-
  Product : Product
  Product1 : Product
  Err : Outport
  wires:
  Minus/1 -> Err/1
  SinValue/1 -> Product/2
  Sin/1 -> Product/1
  Cos/1 -> Product1/1
  CosValue/1 -> Product1/2
  Product/1 -> Minus/1
  Product1/1 -> Minus/2

== system MCU_Input/Input_100us/Encoder_100us/Encoder_100us/EncAngleCal/ErrTwo ==
  Sin : Inport
  Cos : Inport  Port=2
  SinValue : Inport  Port=3
  CosValue : Inport  Port=4
  Minus : Sum  Inputs=+-
  Product : Product
  Product1 : Product
  Err : Outport
  wires:
  Minus/1 -> Err/1
  Product/1 -> Minus/1
  Product1/1 -> Minus/2
  Sin/1 -> Product/1
  CosValue/1 -> Product/2
  SinValue/1 -> Product1/1
  Cos/1 -> Product1/2

== system MCU_Input/Input_100us/Encoder_100us/Encoder_100us/EncAngleCal/FirstCalcStatus ==
  SinValue : Inport
  CosValue : Inport  Port=2
  Enable : EnablePort
  Atan2 : Trigonometry  Operator=atan2
  Constant : Constant  Value=pi  OutDataTypeStr=single
  Constant1 : Constant  OutDataTypeStr=uint8
  Divide : Product  Inputs=*/
  FirstCalAngle : Outport
  FirstCalStatus : Outport  Port=2
  wires:
  Constant/1 -> Divide/2
  Atan2/1 -> Divide/1
  Divide/1 -> FirstCalAngle/1
  SinValue/1 -> Atan2/1
  CosValue/1 -> Atan2/2
  Constant1/1 -> FirstCalStatus/1

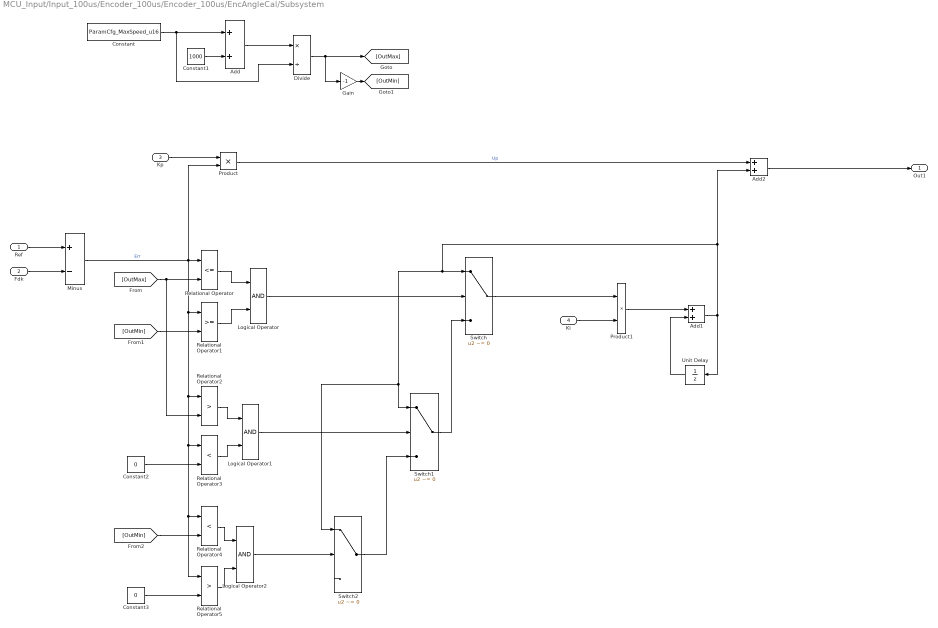
== system MCU_Input/Input_100us/Encoder_100us/Encoder_100us/EncAngleCal/Subsystem ==
  Ref : Inport
  Fdk : Inport  Port=2
  Kp : Inport  Port=3
  Ki : Inport  Port=4
  Add : Sum
  Add1 : Sum
  Add2 : Sum
  Constant : Constant  Value=ParamCfg_MaxSpeed_u16
  Constant1 : Constant  Value=1000  OutDataTypeStr=single
  Constant2 : Constant  Value=0  OutDataTypeStr=single
  Constant3 : Constant  Value=0  OutDataTypeStr=single
  Divide : Product  Inputs=*/
  Gain : Gain  Gain=-1  ParamDataTypeStr=single  OutDataTypeStr=single
  Logical Operator : Logic  AllPortsSameDT=off  OutDataTypeStr=boolean
  Logical Operator1 : Logic  AllPortsSameDT=off  OutDataTypeStr=boolean
  Logical Operator2 : Logic  AllPortsSameDT=off  OutDataTypeStr=boolean
  Minus : Sum  Inputs=+-
  Product : Product
  Product1 : Product
  Relational Operator : RelationalOperator  Operator=<=  OutDataTypeStr=boolean  RndMeth=Simplest  InputSameDT=off
  Relational Operator1 : RelationalOperator  OutDataTypeStr=boolean  RndMeth=Simplest  InputSameDT=off
  Relational Operator2 : RelationalOperator  Operator=>  OutDataTypeStr=boolean  RndMeth=Simplest  InputSameDT=off
  Relational Operator3 : RelationalOperator  Operator=<  OutDataTypeStr=boolean  RndMeth=Simplest  InputSameDT=off
  Relational Operator4 : RelationalOperator  Operator=<  OutDataTypeStr=boolean  RndMeth=Simplest  InputSameDT=off
  Relational Operator5 : RelationalOperator  Operator=>  OutDataTypeStr=boolean  RndMeth=Simplest  InputSameDT=off
  Switch : Switch  Criteria=u2 ~= 0  SaturateOnIntegerOverflow=off  InputSameDT=off
  Switch1 : Switch  Criteria=u2 ~= 0  SaturateOnIntegerOverflow=off  InputSameDT=off
  Switch2 : Switch  Criteria=u2 ~= 0  SaturateOnIntegerOverflow=off  InputSameDT=off
  Unit Delay : UnitDelay  SampleTime=-1  HasFrameUpgradeWarning=on
  Out1 : Outport
  wires:
  Minus/1 -> Product/2, Relational Operator5/1, Relational Operator4/1, Relational Operator3/1, Relational Operator2/1, Relational Operator1/1, Relational Operator/1  "Err"
  Ref/1 -> Minus/1
  Fdk/1 -> Minus/2
  Constant/1 -> Add/1, Divide/2
  Constant1/1 -> Add/2
  Add/1 -> Divide/1
  Divide/1 -> Gain/1, [OutMax]
  Gain/1 -> [OutMin]
  [OutMax] -> Relational Operator2/2, Relational Operator/2
  [OutMin] -> Relational Operator1/2
  Relational Operator/1 -> Logical Operator/1
  Relational Operator1/1 -> Logical Operator/2
  Logical Operator/1 -> Switch/2
  Relational Operator2/1 -> Logical Operator1/1
  Relational Operator3/1 -> Logical Operator1/2
  Constant2/1 -> Relational Operator3/2
  Logical Operator1/1 -> Switch1/2
  Add1/1 -> Unit Delay/1, Switch2/1, Switch1/1, Switch/1, Add2/2
  [OutMin] -> Relational Operator4/2
  Constant3/1 -> Relational Operator5/2
  Relational Operator5/1 -> Logical Operator2/2
  Relational Operator4/1 -> Logical Operator2/1
  Logical Operator2/1 -> Switch2/2
  Kp/1 -> Product/1
  Product/1 -> Add2/1  "Up"
  Switch/1 -> Product1/1
  Ki/1 -> Product1/2
  Product1/1 -> Add1/1
  Unit Delay/1 -> Add1/2
  Add2/1 -> Out1/1
  Switch1/1 -> Switch/3
  Switch2/1 -> Switch1/3

== system MCU_Input/Input_100us/Rotate_100us/RotateCalc/En/Chart/PosDirDispos ==
  dir : Inport  OutDataTypeStr=uint16
  pos : Inport  Port=2
  max_pos : Inport  Port=3
  f : TriggerPort  TriggerType=function-call  VariantControl=(inherit)
      settings: CopyFcn=Stateflow.SLINSF.SimulinkMan.removeBlockPreDeleteFcn  PreDeleteFcn=Stateflow.SLINSF.SimulinkMan.unsafePredeleteFcn
  Minus : Sum  Inputs=+-  OutDataTypeStr=int16
  Switch : Switch  Criteria=u2 ~= 0  SaturateOnIntegerOverflow=off  InputSameDT=off
  tmpPos : Outport
  wires:
  max_pos/1 -> Minus/1
  Switch/1 -> tmpPos/1
  pos/1 -> Minus/2, Switch/1
  Minus/1 -> Switch/3
  dir/1 -> Switch/2

== system MCU_Input/Input_100us/Rotate_100us/RotateCalc/En/Chart/PosLimit ==
  pos : Inport
  MaxPos : Inport  Port=2
  f : TriggerPort  TriggerType=function-call  VariantControl=(inherit)
      settings: CopyFcn=Stateflow.SLINSF.SimulinkMan.removeBlockPreDeleteFcn  PreDeleteFcn=Stateflow.SLINSF.SimulinkMan.unsafePredeleteFcn
  LimitChart : Stateflow chart  TreatAsAtomicUnit=on
  tmpPos : Outport
  wires:
  pos/1 -> LimitChart/1(Pos)
  MaxPos/1 -> LimitChart/2(MaxPos)
  LimitChart/1(tmpPos) -> tmpPos/1

== stateflow chart MCU_Input/Input_100us/Encoder_100us/Encoder_100us/EncCalibCal2 ==
  state Finish [commented out]
  state Normalize [commented out]
    en:
    if(Cnt<AvgCnt)
    SinAmplitude =AmpSin(SinDigitalValue);
    CosAmplitude = AmpCos(CosDigitalValue);
    %SinAmp = SinAmplitude;
    %CosAmp = CosAmplitude;
    SinSum = SinSum + SinDigitalValue;
    CosSum = CosSum + CosDigitalValue;
    Cnt = Cnt+1;
    else
    %求均值
    SinAverage = SinSum/(Cnt);
    CosAverage = CosSum/(Cnt);
    %求幅值倒数
    SinAmplitudeInverse = 1/SinAmplitude;
    CosAmplitudeInverse = 1/CosAmplitude;
    %更新参数，放大十倍写回
    SinAvg = SinAverage*10;
    CosAvg = CosAverage *10;
    SinAmp = SinAmplitude *10;
    CosAmp = CosAmplitude *10;
    SinValue = (SinDigitalValue-SinAverage)*SinAmplitudeInverse;
    CosValue = (CosDigitalValue - CosAverage)*CosAmplitudeInverse;
  state Compensate [commented out]
  state SinAmp = AmpSin(SinRaw) [function]
  state CosAmp = AmpCos(CosRaw) [function]
  (default) -> (junction 118) [commented out]
  (junction 118) -> Finish [commented out]
  (junction 118) -> Normalize [commented out] : [Calib_Stage == NORMALIZE]
  (junction 118) -> Compensate [commented out] : [Calib_Stage == COMPENSATE]
  Normalize -> Finish [commented out]
  (default) -> (junction 94) [commented out]
  (junction 108) -> (junction 117) [commented out] : [Cnt < AvgCnt]{
      | SinAmplitude =AmpSin(SinDigitalValue);
      | CosAmplitude = AmpCos(CosDigitalValue);
      |
      | %SinAmp = SinAmplitude;
      | %CosAmp = CosAmplitude;
      |
      | SinSum = SinSum + SinDigitalValue;
      | CosSum = CosSum + CosDigitalValue;
      | Cnt = Cnt+1;
      | }
  (junction 94) -> (junction 108) [commented out] : [Calib_Stage == NORMALIZE]
  (junction 108) -> (junction 117) [commented out]
  (junction 94) -> (junction 100) [commented out] : {SinSum = 0;
      | CosSum= 0;
      | Cnt = 0;
      | ToFinish = 0;
      | SinValue = (SinDigitalValue-SinAverage)*SinAmplitudeInverse;
      | CosValue = (CosDigitalValue - CosAverage)*CosAmplitudeInverse;
      | }
  (junction 117) -> (junction 95) [commented out] : {
      |     %求均值
      |     SinAverage = SinSum/(Cnt);
      |     CosAverage = CosSum/(Cnt);
      |
      |     %求幅值倒数
      |     SinAmplitudeInverse = 1/SinAmplitude;
      |     CosAmplitudeInverse = 1/CosAmplitude;
      |
      | %更新参数，放大十倍写回
      | SinAvg = SinAverage*10;
      | CosAvg = CosAverage *10;
      | SinAmp = SinAmplitude *10;
      | CosAmp = CosAmplitude *10;
      |
      | SinValue = (SinDigitalValue-SinAverage)*SinAmplitudeInverse;
      | CosValue = (CosDigitalValue - CosAverage)*CosAmplitudeInverse;
      | }
  (junction 100) -> (junction 112) [commented out]
  (junction 95) -> (junction 112) [commented out] : {SinSum = 0;
      | CosSum= 0;
      | Cnt = 0;
      | ToFinish = 0}
  (junction 112) -> (junction 107) [commented out]
  (default) -> (junction 151)
  (junction 151) -> (junction 153) [order 1] : [Calib_Stage == NORMALIZE && ToFinish!=1]
  (junction 151) -> (junction 166) [order 2]
  (junction 153) -> (junction 155)
  (junction 155) -> (junction 157) [order 1] : [Cnt < AvgCnt]
  (junction 155) -> (junction 161) [order 2] : {
      |     %求均值
      |     SinAverage = SinSum/(Cnt);
      |     CosAverage = CosSum/(Cnt);
      |
      |     %求幅值倒数
      |     SinAmplitudeInverse = 1/SinAmplitude;
      |     CosAmplitudeInverse = 1/CosAmplitude;
      |
      | %更新参数，放大十倍写回
      | SinAvg = SinAverage*10;
      | CosAvg = CosAverage *10;
      | SinAmp = SinAmplitude *10;
      | CosAmp = CosAmplitude *10;
      |
      | ToFinish = 1
      |
      | %SinValue = (SinDigitalValue-SinAverage)*SinAmplitudeInverse;
      | %CosValue = (CosDigitalValue - CosAverage)*CosAmplitudeInverse;
      | }
  (junction 157) -> (junction 159) : {
      | SinAmplitude =AmpSin(SinDigitalValue);
      | CosAmplitude = AmpCos(CosDigitalValue);
      |
      | %SinAmp = SinAmplitude;
      | %CosAmp = CosAmplitude;
      |
      | SinSum = SinSum + SinDigitalValue;
      | CosSum = CosSum + CosDigitalValue;
      | Cnt = Cnt+1;
      | }
  (junction 159) -> (junction 161)
  (junction 161) -> (junction 179)
  (junction 166) -> (junction 168) [order 1] : [Calib_Stage==COMPENSATE]
  (junction 166) -> (junction 170) [order 2] : %结束
      | {
      | Cnt=0;
      | SinSum=0
      | CosSum=0;
      | ToFinish=0;
      |
      | %SinAverage = SinAvg*0.1;
      | %CosAverage = CosAvg*0.1;
      |
      | %SinAmplitudeInverse = 1/(SinAmp*0.1);
      | %CosAmplitudeInverse = 1/(CosAmp*0.1);
      | }
  (junction 168) -> (junction 172) : {
      | SinAverage = SinAvg*0.1;
      | CosAverage = CosAvg*0.1;
      |
      | SinAmplitudeInverse = 1/(SinAmp*0.1);
      | CosAmplitudeInverse = 1/(CosAmp*0.1);
      | }
  (junction 172) -> (junction 174)
  (junction 174) -> (junction 176)
  (junction 176) -> (junction 170)
  (junction 179) -> (junction 176)
  (junction 170) -> (junction 182) : {
      | SinValue = (SinDigitalValue-SinAvg*0.1)*1/(SinAmp*0.1);
      | CosValue = (CosDigitalValue - CosAvg*0.1)*1/(CosAmp*0.1);
      | }
  data: SinRaw function_input uint16 size=1; SinAmp function_output single size=1; CosRaw function_input uint16 size=1; CosAmp function_output single; Calib_Stage input uint16; AvgCnt input uint16; CosDigitalValue input uint16; SinDigitalValue input uint16; CosValue output single; SinValue output single; Cnt local uint16 =0; CosSum local uint32 =0; SinSum local uint32 =0; COMPENSATE constant uint16 =2; NORMALIZE constant uint16 =1; SinAverage local single =0; CosAverage local single =0; CosAmplitudeInverse local single =0; SinAmplitudeInverse local single =0; CosAmplitude local single; SinAmplitude local single; CosAvg data_store_memory; SinAvg data_store_memory; SinAmp data_store_memory; CosAmp data_store_memory; ToFinish local uint8 =0
